simulink model "Factorial"  (R2016a)
settings: Solver=FixedStepDiscrete  StartTime=0.0  StopTime=10.0  RelTol=1e-3
settings Model: Creator=Muhammed  LastModifiedBy=Muhammed
settings OptimizationCC: DefaultParameterBehavior=Inlined  InlineInvariantSignals=on  EnableMemcpy=off  OptimizeModelRefInitCode=on  LifeSpan=1
settings DebuggingCC: UnderspecifiedInitializationDetection=Classic  MergeDetectMultiDrivingBlocksExec=none
settings ModelReferenceCC: PropagateSignalLabelsOutOfModel=off
settings RTWCC: SystemTargetFile=ert.tlc  GenCodeOnly=on  TemplateMakefile=ert_default_tmf  GenerateReport=on  IncludeHyperlinkInReport=on  LaunchReport=on  GenerateTraceInfo=on  GenerateTraceReport=on  GenerateTraceReportSl=on  GenerateTraceReportSf=on  GenerateTraceReportEml=on
settings CodeAppCC: ForceParamTrailComments=on  IgnoreCustomStorageClasses=off  OperatorAnnotations=on  SimulinkDataObjDesc=on  SFDataObjDesc=on  MATLABFcnDesc=on  InsertBlockDesc=on  MATLABSourceComments=on
settings ERTTargetCC: GenerateSampleERTMain=on  InlinedParameterPlacement=NonHierarchical  ERTCustomFileTemplate=example_file_process.tlc

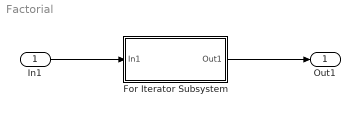
== system Factorial ==
  In1 : Inport
  For Iterator Subsystem : Subsystem  TreatAsAtomicUnit=on
  Out1 : Outport
  wires:
  For Iterator Subsystem/1(Out1) -> Out1/1
  In1/1 -> For Iterator Subsystem/1(In1)

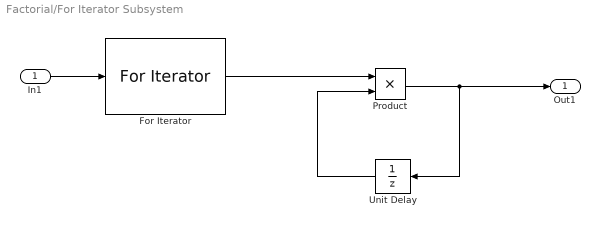
== system Factorial/For Iterator Subsystem ==
  In1 : Inport
  For Iterator : ForIterator  ResetStates=reset  IterationSource=external
  Product : Product  OutDataTypeStr=Inherit: Same as first input
  Unit Delay : UnitDelay  InitialCondition=1  SampleTime=-1
  Out1 : Outport
  wires:
  For Iterator/1 -> Product/1
  In1/1 -> For Iterator/1
  Product/1 -> Out1/1, Unit Delay/1
  Unit Delay/1 -> Product/2
